simulink model "p5"  (R2020a)
settings: Solver=VariableStepAuto  StartTime=0.0  StopTime=10.0  RelTol=1e-3
model workspace (MAT data in the model file):
  C = Simulink.Parameter
  C.Value = 10
  C.DataType = 'auto'
  C.Dimensions = [1 1]
  R = Simulink.Parameter
  R.Value = 10
  R.DataType = 'auto'
  R.Dimensions = [1 1]
undefined symbols (not defined in the file): number, value
settings Model: Creator=007  LastModifiedBy=007

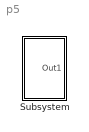
== system p5 ==
  Subsystem : Subsystem

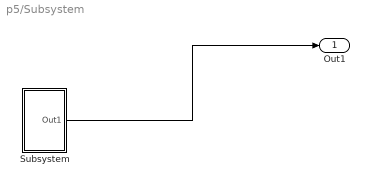
== system p5/Subsystem ==
  Subsystem : Subsystem
  Out1 : Outport
  wires:
  Subsystem/1(Out1) -> Out1/1

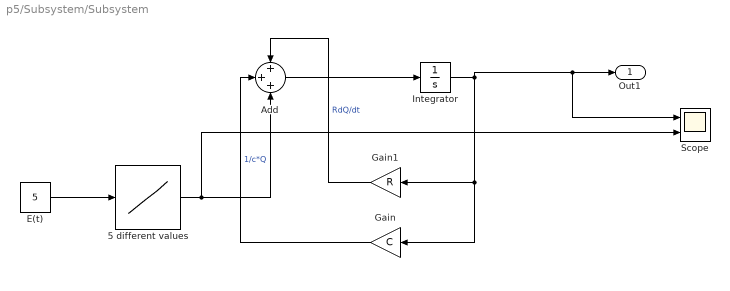
== system p5/Subsystem/Subsystem ==
  5 different values : Lookup_n-D  NumberOfTableDimensions=1  BreakpointsForDimension1=number  Table=value  InternalRulePriority=Speed  RndMeth=Simplest  InputSameDT=on
  Add : Sum  Inputs=+++
  E(t) : Constant  Value=5
  Gain : Gain  Gain=C
  Gain1 : Gain  Gain=R
  Integrator : Integrator
  Scope : Scope  NumInputPorts=2
  Out1 : Outport
  wires:
  Integrator/1 -> Scope/1, Out1/1, Gain/1, Gain1/1
  Gain1/1 -> Add/1  "RdQ/dt"
  5 different values/1 -> Scope/2, Add/3
  Add/1 -> Integrator/1
  Gain/1 -> Add/2  "1/c*Q"
  E(t)/1 -> 5 different values/1
